simulink model "HCO_two_motor_neurons_mod"  (R2022a)
settings: Solver=VariableStepAuto  StartTime=0.0  StopTime=20  RelTol=1e-3
undefined symbols (not defined in the file or in its folder): bar_amp, buff_amp, dfm, dfm_mod, dgsm_g, dhco, dsm, dsm_mod, dsp, dsp_mod, dsyn, dup, dup_mod, gfm, gfm_mod, ghco, gsm, gsm_mod, gsp, gsp_mod, gsyn, gup, gup_mod, Iapp, Iapp_mod, max_torque, noisePwr, rflx_g, sampleTime, sr_gain, X, Y, Z
libraries: sm_lib x12, simulink x8, nesl_utility x8
settings Model: Creator=chris  LastModifiedBy=chris

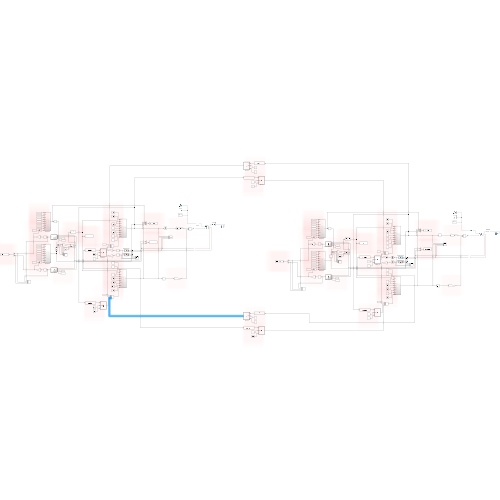
[thumbnail: Simulink's stored preview of the top-level diagram]
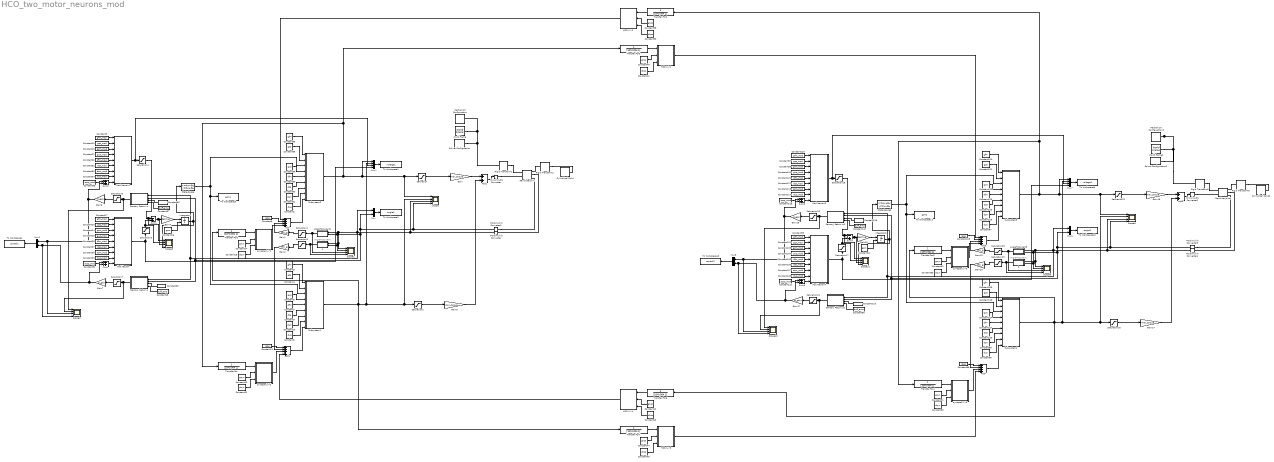
== system HCO_two_motor_neurons_mod ==
  note: AngleToCurrent
  note: AngleToCurrent
  1 : MATLAB Function  TreatAsAtomicUnit=on
  3 : MATLAB Function  TreatAsAtomicUnit=on
  Add{,1,6..7} (4 alike) : Sum  Inputs=++++
  Add2 : Sum
  Add8 : Sum
  AngleToCurrent1 : MATLAB Function  TreatAsAtomicUnit=on
  AngleToCurrent3 : MATLAB Function  TreatAsAtomicUnit=on
  Constant{1..2,87,98} (4 alike) : Constant  Value=dup
  Constant{10,61,88,126} (4 alike) : Constant  Value=dsm
  Constant{21,25,100,104} (4 alike) : Constant  Value=gup_mod
  Constant{22,26,101,105} (4 alike) : Constant  Value=dfm_mod
  Constant{19,23,97,102} (4 alike) : Constant  Value=gsp_mod
  Constant{20,24,99,103} (4 alike) : Constant  Value=gsm_mod
  Constant{27,32,106,112} (4 alike) : Constant  Value=dsp_mod
  Constant{28,33,107,113} (4 alike) : Constant  Value=dsm_mod
  Constant{29,34,108,114} (4 alike) : Constant  Value=dup_mod
  Constant{3,55,109,120} (4 alike) : Constant  Value=gfm
  Constant{8,11,89,128} (4 alike) : Constant  Value=Iapp
  Constant{30,36,110,116} (4 alike) : Constant  Value=bar_amp
  Constant{31,35,111,115} (4 alike) : Constant  Value=Iapp_mod
  Constant{18,37,96,117} (4 alike) : Constant  Value=buff_amp
  Constant{4,56,118,121} (4 alike) : Constant  Value=gsp
  Constant{5,17,95,119} (4 alike) : Constant  Value=gfm_mod
  Constant{12,15,90,93} (4 alike) : Constant  Value=dsyn
  Constant{6,58,122,124} (4 alike) : Constant  Value=gup
  Constant{7,59,123,127} (4 alike) : Constant  Value=dfm
  Constant{9,60,125,129} (4 alike) : Constant  Value=dsp
  Constant{13..14,91..92} (4 alike) : Constant  Value=gsyn
  Constant16 : Constant  Value=gsm
  Constant{38,40,42,44} (4 alike) : Constant  Value=ghco
  Constant{39,41,43,45} (4 alike) : Constant  Value=dhco
  Constant94 : Constant  Value=gsm
  Cylindrical Solid : sm_lib/Body Elements/Cylindrical Solid  GraphicAmbientColor=[0.15 0.15 0.15 1.0]  BasedOnType=Density  CenterOfMass=[0 0 0]  CenterOfMassUnits=m  GraphicDiffuseColor=[0.5 0.5 0.5]  CylinderLength=0.5  CylinderLengthUnits=m  CylinderRadius=0.05  CylinderRadiusUnits=m  Density=1000  DensityUnits=kg/m^3  DoExposeReferenceFrame=on  GraphicEmissiveColor=[0.0 0.0 0.0 1.0]  ExportEntireGeometry=off  SerializedFrames=<Frames/>  MarkerShape=Sphere  MarkerSize=10  GraphicType=FromGeometry  InertiaType=CalculateFromGeometry  Mass=1  MassUnits=kg  MomentsOfInertia=[1 1 1]  MomentsOfInertiaUnits=kg*m^2  GraphicOpacity=1.0  ProductsOfInertia=[0 0 0]  ProductsOfInertiaUnits=kg*m^2  GraphicShininess=75  GraphicSpecularColor=[0.5 0.5 0.5 1.0]  GraphicVisPropType=SimpleVisualProperties
  Cylindrical Solid2 : sm_lib/Body Elements/Cylindrical Solid  GraphicAmbientColor=[0.15 0.15 0.15 1.0]  BasedOnType=Density  CenterOfMass=[0 0 0]  CenterOfMassUnits=m  GraphicDiffuseColor=[0.5 0.5 0.5]  CylinderLength=0.5  CylinderLengthUnits=m  CylinderRadius=0.05  CylinderRadiusUnits=m  Density=1000  DensityUnits=kg/m^3  DoExposeReferenceFrame=on  GraphicEmissiveColor=[0.0 0.0 0.0 1.0]  ExportEntireGeometry=off  SerializedFrames=<Frames/>  MarkerShape=Sphere  MarkerSize=10  GraphicType=FromGeometry  InertiaType=CalculateFromGeometry  Mass=1  MassUnits=kg  MomentsOfInertia=[1 1 1]  MomentsOfInertiaUnits=kg*m^2  GraphicOpacity=1.0  ProductsOfInertia=[0 0 0]  ProductsOfInertiaUnits=kg*m^2  GraphicShininess=75  GraphicSpecularColor=[0.5 0.5 0.5 1.0]  GraphicVisPropType=SimpleVisualProperties
  Gain : Gain  Gain=max_torque
  Gain{1..2,19..20} (4 alike) : Gain  Gain=rflx_g
  Gain14 : Gain  Gain=-max_torque
  Gain15 : Gain  Gain=dgsm_g
  Gain{6..7,16..17} (4 alike) : Gain  Gain=sr_gain
  Gain18 : Gain  Gain=max_torque
  Gain3 : Gain  Gain=-max_torque
  Gain4 : Gain  Gain=dgsm_g
  HCO 1->1 : MATLAB Function  TreatAsAtomicUnit=on
  HCO 1->2 : MATLAB Function  TreatAsAtomicUnit=on
  HCO 1->3 : MATLAB Function  TreatAsAtomicUnit=on
  HCO 1->4 : MATLAB Function  TreatAsAtomicUnit=on
  Integrator : Integrator  InitialConditionSource=external
  Integrator2 : Integrator  InitialConditionSource=external
  Mechanism Configuration : sm_lib/Utilities/Mechanism Configuration  UniformGravity=Constant  GravityVector=[0 0 -9.80665]  GravityUnits=m/s^2  LinearizationDelta=0.001  JointModeTransitionNonlinearIterations=2
  Mechanism Configuration2 : sm_lib/Utilities/Mechanism Configuration  UniformGravity=Constant  GravityVector=[0 0 -9.80665]  GravityUnits=m/s^2  LinearizationDelta=0.001  JointModeTransitionNonlinearIterations=2
  Mod Neuron : Subsystem
  Mod Neuron1 : Subsystem
  Mod Neuron4 : Subsystem
  Mod Neuron5 : Subsystem
  Mux{,2,6,8} (4 alike) : Mux  Inputs=2
  Mux1 : Mux
  Mux7 : Mux
  PS-Simulink Converter{,1,4..5} (4 alike) : nesl_utility/PS-Simulink Converter  PhysicalDomain=network_engine_domain  SubClassName=ps_output  LeftPortType=input  RightPortType=output  PseudoPeriodic=off  Frequencies=[]  VectorFormat=inherit  Unit=inherit  AffineConversion=off
      settings: SourceProductBaseCode=SS,PW,VE
  Revolute Joint : sm_lib/Joints/Revolute Joint  JointMode=Normal  SenseConstraintForce=off  SenseConstraintForceX=off  SenseConstraintForceY=off  SenseConstraintForceZ=off  SenseConstraintTorque=off  SenseConstraintTorqueX=off  SenseConstraintTorqueY=off  SenseConstraintTorqueZ=off  SenseTotalForce=off  SenseTotalForceX=off  SenseTotalForceY=off  SenseTotalForceZ=off  SenseTotalTorque=off  SenseTotalTorqueX=off  SenseTotalTorqueY=off  SenseTotalTorqueZ=off  CompositeWrenchDir=FollowerOnBase  CompositeWrenchFrame=BaseFrame  EquilibriumPosition=0  EquilibriumPositionUnits=deg  SpringStiffness=0.0  SpringStiffnessUnits=N*m/deg  DampingCoefficient=0.01  DampingCoefficientUnits=N*m/(deg/s)  TorqueActuationMode=InputTorque  MotionActuationMode=ComputedMotion  SensePosition=on  SenseVelocity=on  SenseAcceleration=off  SenseTorqueForce=off  SenseLowerLimitTorqueForce=off  SenseUpperLimitTorqueForce=off  LowerLimitSpecify=off  LowerLimitBound=-90  LowerLimitBoundUnits=deg  LowerLimitStiffness=1e4  LowerLimitStiffnessUnits=N*m/deg  LowerLimitDamping=10  LowerLimitDampingUnits=N*m/(deg/s)  LowerLimitTransitionRegionWidth=0.1  LowerLimitTransitionRegionWidthUnits=deg  UpperLimitSpecify=off  UpperLimitBound=90  UpperLimitBoundUnits=deg  UpperLimitStiffness=1e4  UpperLimitStiffnessUnits=N*m/deg  UpperLimitDamping=10  UpperLimitDampingUnits=N*m/(deg/s)  UpperLimitTransitionRegionWidth=0.1  UpperLimitTransitionRegionWidthUnits=deg  PositionTargetSpecify=on  PositionTargetPriority=High  PositionTargetValue=20  PositionTargetValueUnits=deg  VelocityTargetSpecify=off  VelocityTargetPriority=High  VelocityTargetValue=0  VelocityTargetValueUnits=deg/s
  Revolute Joint2 : sm_lib/Joints/Revolute Joint  JointMode=Normal  SenseConstraintForce=off  SenseConstraintForceX=off  SenseConstraintForceY=off  SenseConstraintForceZ=off  SenseConstraintTorque=off  SenseConstraintTorqueX=off  SenseConstraintTorqueY=off  SenseConstraintTorqueZ=off  SenseTotalForce=off  SenseTotalForceX=off  SenseTotalForceY=off  SenseTotalForceZ=off  SenseTotalTorque=off  SenseTotalTorqueX=off  SenseTotalTorqueY=off  SenseTotalTorqueZ=off  CompositeWrenchDir=FollowerOnBase  CompositeWrenchFrame=BaseFrame  EquilibriumPosition=0  EquilibriumPositionUnits=deg  SpringStiffness=0.0  SpringStiffnessUnits=N*m/deg  DampingCoefficient=0.01  DampingCoefficientUnits=N*m/(deg/s)  TorqueActuationMode=InputTorque  MotionActuationMode=ComputedMotion  SensePosition=on  SenseVelocity=on  SenseAcceleration=off  SenseTorqueForce=off  SenseLowerLimitTorqueForce=off  SenseUpperLimitTorqueForce=off  LowerLimitSpecify=off  LowerLimitBound=-90  LowerLimitBoundUnits=deg  LowerLimitStiffness=1e4  LowerLimitStiffnessUnits=N*m/deg  LowerLimitDamping=10  LowerLimitDampingUnits=N*m/(deg/s)  LowerLimitTransitionRegionWidth=0.1  LowerLimitTransitionRegionWidthUnits=deg  UpperLimitSpecify=off  UpperLimitBound=90  UpperLimitBoundUnits=deg  UpperLimitStiffness=1e4  UpperLimitStiffnessUnits=N*m/deg  UpperLimitDamping=10  UpperLimitDampingUnits=N*m/(deg/s)  UpperLimitTransitionRegionWidth=0.1  UpperLimitTransitionRegionWidthUnits=deg  PositionTargetSpecify=on  PositionTargetPriority=High  PositionTargetValue=20  PositionTargetValueUnits=deg  VelocityTargetSpecify=off  VelocityTargetPriority=High  VelocityTargetValue=0  VelocityTargetValueUnits=deg/s
  Rigid Transform1 : sm_lib/Frames and Transforms/Rigid Transform  TranslationMethod=None  TranslationStandardOffset=0.25  TranslationLengthUnit=m  TranslationStandardAxis=+X  TranslationCartesianOffset=[0 0 0]  TranslationROffset=0  TranslationROffsetUnits=m  TranslationZOffset=0  TranslationZOffsetUnits=m  TranslationThetaOffset=0  TranslationThetaOffsetUnits=deg  RotationMethod=RotationSequence  RotationAngleUnits=deg  RotationStandardAxis=+Y  RotationAngle=90  RotationArbitraryAxis=[0 0 1]  FollAlignAxisA=+X  BaseAlignAxisA=+Y  FollAlignAxisB=+Y  BaseAlignAxisB=+Z  RotationSequenceAxes=FollowerAxes  RotationSequence=XYX  RotationSequenceAngles=[0 90 90]  RotationSequenceAnglesUnits=deg  RotationMatrix=[1 0 0; 0 1 0; 0 0 1]
  Rigid Transform2 : sm_lib/Frames and Transforms/Rigid Transform  TranslationMethod=StandardAxis  TranslationStandardOffset=.25  TranslationLengthUnit=m  TranslationStandardAxis=+X  TranslationCartesianOffset=[0 0 0]  TranslationROffset=0  TranslationROffsetUnits=m  TranslationZOffset=0  TranslationZOffsetUnits=m  TranslationThetaOffset=0  TranslationThetaOffsetUnits=deg  RotationMethod=RotationSequence  RotationAngleUnits=deg  RotationStandardAxis=+Z  RotationAngle=90  RotationArbitraryAxis=[0 0 1]  FollAlignAxisA=+X  BaseAlignAxisA=+Y  FollAlignAxisB=+Y  BaseAlignAxisB=+Z  RotationSequenceAxes=FollowerAxes  RotationSequence=XYX  RotationSequenceAngles=[0 90 0]  RotationSequenceAnglesUnits=deg  RotationMatrix=[1 0 0; 0 1 0; 0 0 1]
  Rigid Transform5 : sm_lib/Frames and Transforms/Rigid Transform  TranslationMethod=None  TranslationStandardOffset=0.25  TranslationLengthUnit=m  TranslationStandardAxis=+X  TranslationCartesianOffset=[0 0 0]  TranslationROffset=0  TranslationROffsetUnits=m  TranslationZOffset=0  TranslationZOffsetUnits=m  TranslationThetaOffset=0  TranslationThetaOffsetUnits=deg  RotationMethod=RotationSequence  RotationAngleUnits=deg  RotationStandardAxis=+Y  RotationAngle=90  RotationArbitraryAxis=[0 0 1]  FollAlignAxisA=+X  BaseAlignAxisA=+Y  FollAlignAxisB=+Y  BaseAlignAxisB=+Z  RotationSequenceAxes=FollowerAxes  RotationSequence=XYX  RotationSequenceAngles=[0 90 90]  RotationSequenceAnglesUnits=deg  RotationMatrix=[1 0 0; 0 1 0; 0 0 1]
  Rigid Transform6 : sm_lib/Frames and Transforms/Rigid Transform  TranslationMethod=StandardAxis  TranslationStandardOffset=.25  TranslationLengthUnit=m  TranslationStandardAxis=+X  TranslationCartesianOffset=[0 0 0]  TranslationROffset=0  TranslationROffsetUnits=m  TranslationZOffset=0  TranslationZOffsetUnits=m  TranslationThetaOffset=0  TranslationThetaOffsetUnits=deg  RotationMethod=RotationSequence  RotationAngleUnits=deg  RotationStandardAxis=+Z  RotationAngle=90  RotationArbitraryAxis=[0 0 1]  FollAlignAxisA=+X  BaseAlignAxisA=+Y  FollAlignAxisB=+Y  BaseAlignAxisB=+Z  RotationSequenceAxes=FollowerAxes  RotationSequence=XYX  RotationSequenceAngles=[0 90 0]  RotationSequenceAnglesUnits=deg  RotationMatrix=[1 0 0; 0 1 0; 0 0 1]
  Saturation{,1..7,16..23} (16 alike) : Saturate  UpperLimit=1.0  LowerLimit=0.0
  Scope{,1..3,8..11} (8 alike) : Scope  NumInputPorts=4
  Sensory Return m : MATLAB Function  TreatAsAtomicUnit=on
  Sensory Return m2 : MATLAB Function  TreatAsAtomicUnit=on
  Sensory Return p : MATLAB Function  TreatAsAtomicUnit=on
  Sensory Return p2 : MATLAB Function  TreatAsAtomicUnit=on
  Simulink-PS Converter : nesl_utility/Simulink-PS Converter  PhysicalDomain=network_engine_domain  SubClassName=ps_input  LeftPortType=input  RightPortType=output  PseudoPeriodic=off  Frequencies=[]  NoiseDistribution=none  NoiseParameters=[]  Unit=1  AffineConversion=off  FilteringAndDerivatives=provide  SimscapeFilterOrder=1  InputFilterTimeConstant=0.001  UdotUserProvided=0
      settings: SourceProductBaseCode=SS,PW,VE
  Simulink-PS Converter2 : nesl_utility/Simulink-PS Converter  PhysicalDomain=network_engine_domain  SubClassName=ps_input  LeftPortType=input  RightPortType=output  PseudoPeriodic=off  Frequencies=[]  NoiseDistribution=none  NoiseParameters=[]  Unit=1  AffineConversion=off  FilteringAndDerivatives=provide  SimscapeFilterOrder=1  InputFilterTimeConstant=0.001  UdotUserProvided=0
      settings: SourceProductBaseCode=SS,PW,VE
  Solver Configuration : nesl_utility/Solver Configuration  PhysicalDomain=network_engine_domain  SubClassName=solver  LeftPortType=input  RightPortType=generic  Tones=[]  Harmonics=[]  SimulateNoise=off  Profile=off  UseLocalSampling=off  EnableSwitchedLinearOptims=on  FrequencyDomain=off  UseCCode=off  RelTol=0.001  AbsTol=1e-06  MinStep=1e-09  ToWorkspace=off  RevertToSquareIcSolve=off  NumHomotopyIterations=100  PhasorMode=off  PhasorModeNumHarmonics=1  IndexReductionMethod=DerivativeReplacement  DoDC=off  ResidualTolerance=1e-09  UseLocalSolver=off  LocalSolverChoice=NE_BACKWARD_EULER_ADVANCER  LocalSolverSampleTime=0.001  DoFixedCost=off  MaxNonlinIter=3  MaxModeIter=2  ComputeImpulses=off  ImpulseIterations=2  LinearAlgebra=auto  LinearAlgebraNumThread=0  EquationFormulation=NE_TIME_EF  DelaysMemoryBudget=1024  AutomaticFiltering=on  FilteringTimeConstant=0.001  PartitionStorageMethod=AS_NEEDED  PartitionMemoryBudget=1024  PartitionMethod=ROBUST
      settings: SourceProductBaseCode=SS,PW,VE
  Solver Configuration2 : nesl_utility/Solver Configuration  PhysicalDomain=network_engine_domain  SubClassName=solver  LeftPortType=input  RightPortType=generic  Tones=[]  Harmonics=[]  SimulateNoise=off  Profile=off  UseLocalSampling=off  EnableSwitchedLinearOptims=on  FrequencyDomain=off  UseCCode=off  RelTol=0.001  AbsTol=1e-06  MinStep=1e-09  ToWorkspace=off  RevertToSquareIcSolve=off  NumHomotopyIterations=100  PhasorMode=off  PhasorModeNumHarmonics=1  IndexReductionMethod=DerivativeReplacement  DoDC=off  ResidualTolerance=1e-09  UseLocalSolver=off  LocalSolverChoice=NE_BACKWARD_EULER_ADVANCER  LocalSolverSampleTime=0.001  DoFixedCost=off  MaxNonlinIter=3  MaxModeIter=2  ComputeImpulses=off  ImpulseIterations=2  LinearAlgebra=auto  LinearAlgebraNumThread=0  EquationFormulation=NE_TIME_EF  DelaysMemoryBudget=1024  AutomaticFiltering=on  FilteringTimeConstant=0.001  PartitionStorageMethod=AS_NEEDED  PartitionMemoryBudget=1024  PartitionMethod=ROBUST
      settings: SourceProductBaseCode=SS,PW,VE
  State-Space : StateSpace  A=-10  B=10  D=0  InitialCondition=gsm
  State-Space2 : StateSpace  A=-10  B=10  D=0  InitialCondition=gsm
  Subsystem1 : Subsystem
  Subsystem4 : Subsystem
  Subsystem5 : Subsystem
  Subsystem6 : Subsystem
  Sum{,2,6,8} (4 alike) : Sum
  Sum1 : Sum  Inputs=-+
  Sum7 : Sum  Inputs=-+
  To Workspace1 : ToWorkspace  VariableName=voltage1  SaveFormat=Structure With Time  SampleTime=sampleTime
  To Workspace10 : ToWorkspace  VariableName=angle2  SaveFormat=Structure With Time  SampleTime=sampleTime
  To Workspace11 : ToWorkspace  VariableName=gsm2  SaveFormat=Structure With Time  SampleTime=sampleTime
  To Workspace12 : ToWorkspace  VariableName=control2  SaveFormat=Structure With Time  SampleTime=sampleTime
  To Workspace2 : ToWorkspace  VariableName=angle1  SaveFormat=Structure With Time  SampleTime=sampleTime
  To Workspace3 : ToWorkspace  VariableName=gsm1  SaveFormat=Structure With Time  SampleTime=sampleTime
  To Workspace4 : ToWorkspace  VariableName=control1  SaveFormat=Structure With Time  SampleTime=sampleTime
  To Workspace9 : ToWorkspace  VariableName=voltage2  SaveFormat=Structure With Time  SampleTime=sampleTime
  Transfer Fcn{,1..7} (8 alike) : TransferFcn  Denominator=[10*0.004 1]
  World Frame : sm_lib/Frames and Transforms/World Frame
  World Frame2 : sm_lib/Frames and Transforms/World Frame
  synapse 1->1 : MATLAB Function  TreatAsAtomicUnit=on
  synapse 1->2 : MATLAB Function  TreatAsAtomicUnit=on
  synapse 1->5 : MATLAB Function  TreatAsAtomicUnit=on
  synapse 1->6 : MATLAB Function  TreatAsAtomicUnit=on
  wires:
  Subsystem6/1(V) -> Scope/1, Saturation/1, Mux1/1, Transfer Fcn3/1, Transfer Fcn/1
  Constant60/1 -> Subsystem6/6(dsp)
  Constant1/1 -> Subsystem6/8(dup)
  Constant59/1 -> Subsystem6/5(dfm)
  Constant61/1 -> Subsystem6/7(dsm)
  Constant56/1 -> Subsystem6/2(gsp)
  Constant58/1 -> Subsystem6/4(gup)
  Constant55/1 -> Subsystem6/1(gfm)
  Saturation/1 -> Gain/1
  Add/1 -> Subsystem6/9(Iapp)
  Mux/1 -> To Workspace2/1
  PS-Simulink Converter1/1 -> Scope/4, Mux/2, Scope1/2, 1/2(du), AngleToCurrent1/2(du), Sensory Return m/2(du), Sensory Return p/2(du)
  Constant9/1 -> Subsystem1/6(dsp)
  Constant11/1 -> Add1/1
  Constant10/1 -> Subsystem1/7(dsm)
  Constant3/1 -> Subsystem1/1(gfm)
  Constant4/1 -> Subsystem1/2(gsp)
  Constant7/1 -> Subsystem1/5(dfm)
  Add1/1 -> Subsystem1/9(Iapp)
  Constant6/1 -> Subsystem1/4(gup)
  Constant2/1 -> Subsystem1/8(dup)
  Gain2/1 -> Add1/2
  Subsystem1/1(V) -> Transfer Fcn1/1, Transfer Fcn7/1, Saturation2/1, Scope/2, Mux1/2
  Saturation2/1 -> Gain3/1
  Add2/1 -> Simulink-PS Converter/1
  Gain/1 -> Add2/1
  Gain3/1 -> Add2/2
  synapse 1->2/1(I) -> Add1/3
  Transfer Fcn/1 -> synapse 1->2/1(V)
  Transfer Fcn1/1 -> synapse 1->1/1(V)
  Constant13/1 -> synapse 1->2/2(gsyn)
  Constant12/1 -> synapse 1->2/3(d)
  Constant15/1 -> synapse 1->1/3(d)
  Constant14/1 -> synapse 1->1/2(gsyn)
  Mux1/1 -> To Workspace1/1
  Sum/1 -> Mod Neuron/9(Iapp)
  Constant30/1 -> Sensory Return p/3(bar_amp)
  Constant17/1 -> Mod Neuron/1(gfm)
  Constant23/1 -> Mod Neuron/2(gsp)
  Constant31/1 -> Sum/1
  Constant28/1 -> Mod Neuron/7(dsm)
  Constant26/1 -> Mod Neuron/5(dfm)
  Constant27/1 -> Mod Neuron/6(dsp)
  Constant24/1 -> Mod Neuron/3(gsm)
  Constant25/1 -> Mod Neuron/4(gup)
  Constant29/1 -> Mod Neuron/8(dup)
  PS-Simulink Converter/1 -> Scope/3, Scope1/1, 1/1(u), AngleToCurrent1/1(u), Sensory Return m/1(u), Sensory Return p/1(u), Mux/1
  Constant16/1 -> Integrator/2
  Mod Neuron/1(V) -> Saturation3/1, Mux1/4
  Saturation4/1 -> Scope3/1, Sum1/1
  Saturation3/1 -> Scope3/2, Sum1/2
  Integrator/1 -> State-Space/1, Scope3/4
  State-Space/1 -> Subsystem6/3(gsm), Subsystem1/3(gsm), To Workspace3/1
  Gain4/1 -> Integrator/1
  Sum1/1 -> Scope3/3, Gain4/1
  Sum2/1 -> Mod Neuron1/9(Iapp)
  Constant22/1 -> Mod Neuron1/5(dfm)
  Constant35/1 -> Sum2/1
  Constant21/1 -> Mod Neuron1/4(gup)
  Constant32/1 -> Mod Neuron1/6(dsp)
  Constant20/1 -> Mod Neuron1/3(gsm)
  Constant33/1 -> Mod Neuron1/7(dsm)
  Constant5/1 -> Mod Neuron1/1(gfm)
  Constant19/1 -> Mod Neuron1/2(gsp)
  Constant34/1 -> Mod Neuron1/8(dup)
  Constant36/1 -> Sensory Return m/3(bar_amp)
  Sensory Return m/1(y) -> Scope2/1, Saturation6/1
  Mod Neuron1/1(V) -> Mux1/3, Saturation4/1
  Mux2/1 -> To Workspace4/1
  Saturation1/1 -> Gain1/1
  Saturation5/1 -> Gain2/1
  Gain6/1 -> Scope2/3, Mux2/1, Sum2/2
  Sensory Return p/1(y) -> Scope2/2, Saturation7/1
  Gain7/1 -> Mux2/2, Scope2/4, Sum/2
  AngleToCurrent1/1(y) -> Saturation1/1, Scope1/3
  1/1(y) -> Scope1/4, Saturation5/1
  Saturation6/1 -> Gain6/1
  Saturation7/1 -> Gain7/1
  Constant18/1 -> Sensory Return p/4(buff_amp)
  Constant37/1 -> Sensory Return m/4(buff_amp)
  Constant120/1 -> Subsystem5/1(gfm)
  Constant105/1 -> Mod Neuron4/5(dfm)
  Constant121/1 -> Subsystem5/2(gsp)
  Saturation22/1 -> Gain18/1
  Constant122/1 -> Subsystem5/4(gup)
  Mux6/1 -> To Workspace10/1
  Constant126/1 -> Subsystem5/7(dsm)
  Add6/1 -> Subsystem5/9(Iapp)
  Constant118/1 -> Subsystem4/2(gsp)
  State-Space2/1 -> To Workspace11/1, Subsystem4/3(gsm), Subsystem5/3(gsm)
  Gain20/1 -> Add7/2
  Constant89/1 -> Add7/1
  Transfer Fcn4/1 -> synapse 1->6/1(V)
  Constant90/1 -> synapse 1->6/3(d)
  Constant92/1 -> synapse 1->5/2(gsyn)
  Constant91/1 -> synapse 1->6/2(gsyn)
  PS-Simulink Converter5/1 -> Sensory Return p2/2(du), Sensory Return m2/2(du), AngleToCurrent3/2(du), 3/2(du), Scope9/2, Mux6/2, Scope8/4
  Sum6/1 -> Mod Neuron4/9(Iapp)
  Constant93/1 -> synapse 1->5/3(d)
  Saturation16/1 -> Gain14/1
  Saturation17/1 -> Sum7/2, Scope11/2
  Constant123/1 -> Subsystem5/5(dfm)
  Gain14/1 -> Add8/2
  Constant124/1 -> Subsystem4/4(gup)
  Constant102/1 -> Mod Neuron4/2(gsp)
  Constant104/1 -> Mod Neuron4/4(gup)
  Constant111/1 -> Sum6/1
  Constant103/1 -> Mod Neuron4/3(gsm)
  Mux7/1 -> To Workspace9/1
  Constant110/1 -> Sensory Return p2/3(bar_amp)
  Constant127/1 -> Subsystem4/5(dfm)
  Integrator2/1 -> Scope11/4, State-Space2/1
  Constant94/1 -> Integrator2/2
  Constant108/1 -> Mod Neuron4/8(dup)
  PS-Simulink Converter4/1 -> Mux6/1, Sensory Return p2/1(u), Sensory Return m2/1(u), AngleToCurrent3/1(u), 3/1(u), Scope9/1, Scope8/3
  Subsystem4/1(V) -> Transfer Fcn6/1, Mux7/2, Scope8/2, Saturation16/1, Transfer Fcn5/1
  Sensory Return m2/1(y) -> Saturation20/1, Scope10/1
  Constant97/1 -> Mod Neuron5/2(gsp)
  Constant116/1 -> Sensory Return m2/3(bar_amp)
  Gain15/1 -> Integrator2/1
  Sum7/1 -> Gain15/1, Scope11/3
  Subsystem5/1(V) -> Transfer Fcn2/1, Transfer Fcn4/1, Mux7/1, Saturation22/1, Scope8/1
  Add8/1 -> Simulink-PS Converter2/1
  Constant109/1 -> Subsystem4/1(gfm)
  Constant98/1 -> Subsystem4/8(dup)
  Constant101/1 -> Mod Neuron5/5(dfm)
  Add7/1 -> Subsystem4/9(Iapp)
  Sensory Return p2/1(y) -> Saturation21/1, Scope10/2
  Gain16/1 -> Sum8/2, Mux8/1, Scope10/3
  Constant115/1 -> Sum8/1
  Saturation23/1 -> Gain19/1
  Constant99/1 -> Mod Neuron5/3(gsm)
  Constant106/1 -> Mod Neuron4/6(dsp)
  Saturation19/1 -> Gain20/1
  Mod Neuron5/1(V) -> Saturation18/1, Mux7/3
  Constant113/1 -> Mod Neuron5/7(dsm)
  Constant114/1 -> Mod Neuron5/8(dup)
  Constant119/1 -> Mod Neuron5/1(gfm)
  Mux8/1 -> To Workspace12/1
  AngleToCurrent3/1(y) -> Scope9/3, Saturation23/1
  Saturation20/1 -> Gain16/1
  Gain17/1 -> Sum6/2, Scope10/4, Mux8/2
  Constant129/1 -> Subsystem4/6(dsp)
  Saturation18/1 -> Sum7/1, Scope11/1
  synapse 1->6/1(I) -> Add7/3
  Constant96/1 -> Sensory Return p2/4(buff_amp)
  Transfer Fcn5/1 -> synapse 1->5/1(V)
  Constant100/1 -> Mod Neuron5/4(gup)
  Constant107/1 -> Mod Neuron4/7(dsm)
  Saturation21/1 -> Gain17/1
  Constant112/1 -> Mod Neuron5/6(dsp)
  Gain18/1 -> Add8/1
  Mod Neuron4/1(V) -> Mux7/4, Saturation17/1
  Sum8/1 -> Mod Neuron5/9(Iapp)
  Constant88/1 -> Subsystem4/7(dsm)
  Constant95/1 -> Mod Neuron4/1(gfm)
  3/1(y) -> Saturation19/1, Scope9/4
  Constant117/1 -> Sensory Return m2/4(buff_amp)
  Constant87/1 -> Subsystem5/8(dup)
  Constant125/1 -> Subsystem5/6(dsp)
  Transfer Fcn7/1 -> HCO 1->3/1(V)
  Constant44/1 -> HCO 1->3/2(gsyn)
  Constant45/1 -> HCO 1->3/3(d)
  Transfer Fcn6/1 -> HCO 1->4/1(V)
  Constant43/1 -> HCO 1->4/3(d)
  Constant42/1 -> HCO 1->4/2(gsyn)
  Transfer Fcn3/1 -> HCO 1->1/1(V)
  Constant40/1 -> HCO 1->1/2(gsyn)
  Constant41/1 -> HCO 1->1/3(d)
  Transfer Fcn2/1 -> HCO 1->2/1(V)
  Constant39/1 -> HCO 1->2/3(d)
  Constant38/1 -> HCO 1->2/2(gsyn)
  synapse 1->1/1(I) -> Add/4
  Gain1/1 -> Add/3
  Constant8/1 -> Add/2
  HCO 1->2/1(I) -> Add/1
  Gain19/1 -> Add6/3
  synapse 1->5/1(I) -> Add6/4
  Constant128/1 -> Add6/2
  HCO 1->1/1(I) -> Add6/1
  HCO 1->3/1(I) -> Add7/4
  HCO 1->4/1(I) -> Add1/4
  connections:
  Solver Configuration/RConn1 -- Mechanism Configuration/RConn1 -- World Frame/RConn1 -- Rigid Transform1/LConn1
  Rigid Transform1/RConn1 -- Revolute Joint/LConn1
  Simulink-PS Converter/RConn1 -- Revolute Joint/LConn2
  Rigid Transform2/RConn1 -- Cylindrical Solid/RConn1
  Rigid Transform2/LConn1 -- Revolute Joint/RConn1
  Revolute Joint/RConn2 -- PS-Simulink Converter/LConn1
  PS-Simulink Converter1/LConn1 -- Revolute Joint/RConn3
  Mechanism Configuration2/RConn1 -- Rigid Transform5/LConn1 -- Solver Configuration2/RConn1 -- World Frame2/RConn1
  Simulink-PS Converter2/RConn1 -- Revolute Joint2/LConn2
  PS-Simulink Converter5/LConn1 -- Revolute Joint2/RConn3
  Rigid Transform5/RConn1 -- Revolute Joint2/LConn1
  Revolute Joint2/RConn2 -- PS-Simulink Converter4/LConn1
  Rigid Transform6/LConn1 -- Revolute Joint2/RConn1
  Rigid Transform6/RConn1 -- Cylindrical Solid2/RConn1

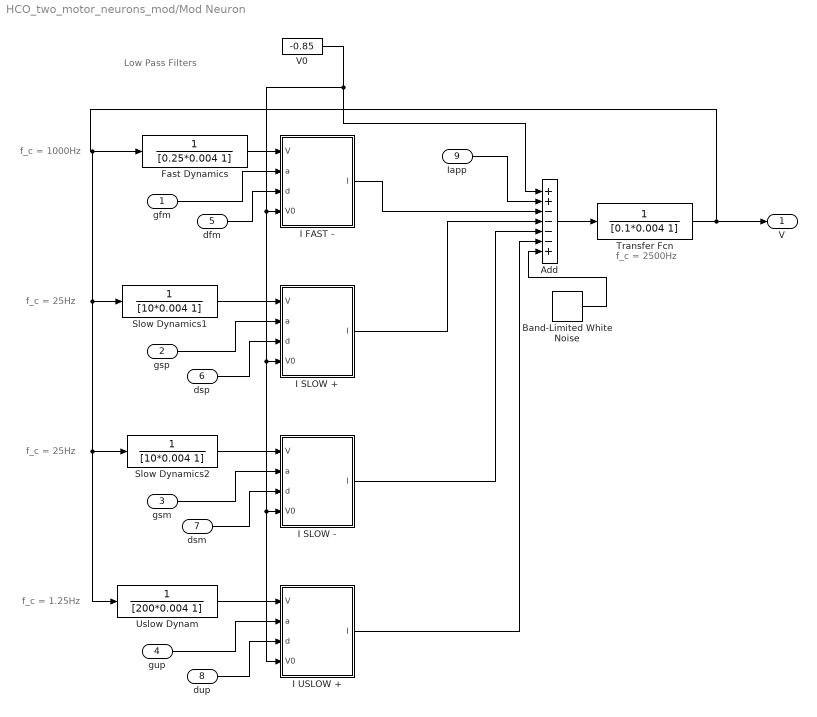
== system HCO_two_motor_neurons_mod/Mod Neuron ==
  note: f_c = 2500Hz
  note: f_c = 1.25Hz
  note: f_c = 25Hz
  note: f_c = 1000Hz
  note: Low Pass Filters
  note: f_c = 25Hz
  gfm : Inport
  gsp : Inport  Port=2
  gsm : Inport  Port=3
  gup : Inport  Port=4
  dfm : Inport  Port=5
  dsp : Inport  Port=6
  dsm : Inport  Port=7
  dup : Inport  Port=8
  Iapp : Inport  Port=9
  Add : Sum  Inputs=++----+
  Band-Limited White Noise : simulink/Sources/Band-Limited White Noise  Cov=[0.0]  Ts=0.1  seed=[23341]
  Fast Dynamics : TransferFcn  Denominator=[0.25*0.004 1]
  I FAST - : MATLAB Function  TreatAsAtomicUnit=on
  I SLOW + : MATLAB Function  TreatAsAtomicUnit=on
  I SLOW - : MATLAB Function  TreatAsAtomicUnit=on
  I USLOW + : MATLAB Function  TreatAsAtomicUnit=on
  Slow Dynamics1 : TransferFcn  Denominator=[10*0.004 1]
  Slow Dynamics2 : TransferFcn  Denominator=[10*0.004 1]
  Transfer Fcn : TransferFcn  Denominator=[0.1*0.004 1]
  Uslow Dynam : TransferFcn  Denominator=[200*0.004 1]
  V0 : Constant  Value=-0.85
  V : Outport
  wires:
  dup/1 -> I USLOW +/3(d)
  gsm/1 -> I SLOW -/2(a)
  dsm/1 -> I SLOW -/3(d)
  gup/1 -> I USLOW +/2(a)
  Iapp/1 -> Add/2
  Uslow Dynam/1 -> I USLOW +/1(V)
  Add/1 -> Transfer Fcn/1
  Slow Dynamics1/1 -> I SLOW +/1(V)
  Slow Dynamics2/1 -> I SLOW -/1(V)
  I FAST -/1(I) -> Add/3
  I USLOW +/1(I) -> Add/6
  V0/1 -> I USLOW +/4(V0), I SLOW -/4(V0), I SLOW +/4(V0), I FAST -/4(V0), Add/1
  dsp/1 -> I SLOW +/3(d)
  gsp/1 -> I SLOW +/2(a)
  dfm/1 -> I FAST -/3(d)
  gfm/1 -> I FAST -/2(a)
  Fast Dynamics/1 -> I FAST -/1(V)
  I SLOW -/1(I) -> Add/5
  Transfer Fcn/1 -> V/1, Uslow Dynam/1, Slow Dynamics2/1, Slow Dynamics1/1, Fast Dynamics/1
  I SLOW +/1(I) -> Add/4
  Band-Limited White Noise/1 -> Add/7

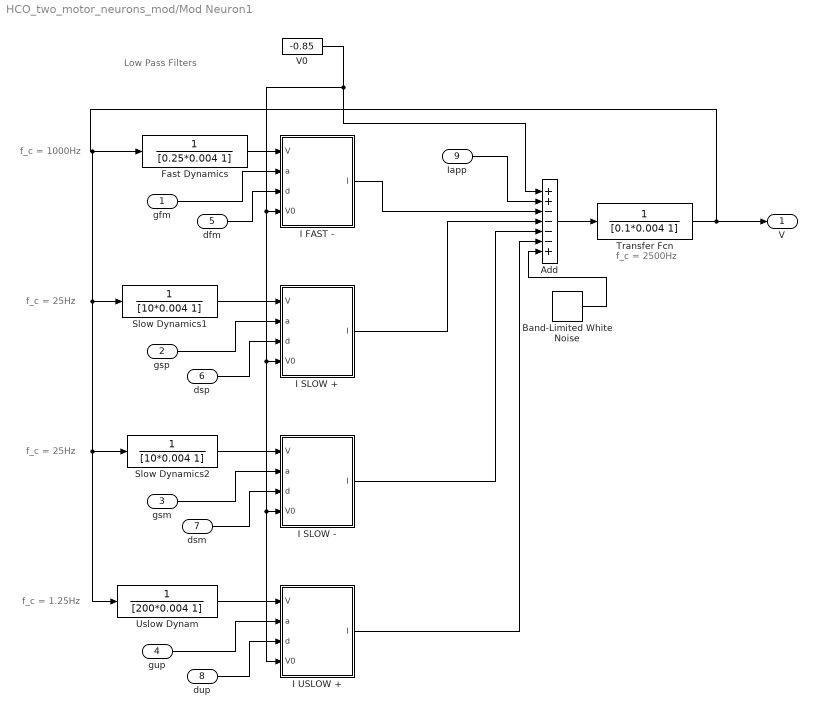
== system HCO_two_motor_neurons_mod/Mod Neuron1 ==
  note: f_c = 2500Hz
  note: f_c = 1.25Hz
  note: f_c = 25Hz
  note: f_c = 1000Hz
  note: Low Pass Filters
  note: f_c = 25Hz
  gfm : Inport
  gsp : Inport  Port=2
  gsm : Inport  Port=3
  gup : Inport  Port=4
  dfm : Inport  Port=5
  dsp : Inport  Port=6
  dsm : Inport  Port=7
  dup : Inport  Port=8
  Iapp : Inport  Port=9
  Add : Sum  Inputs=++----+
  Band-Limited White Noise : simulink/Sources/Band-Limited White Noise  Cov=[0.0]  Ts=0.1  seed=[23341]
  Fast Dynamics : TransferFcn  Denominator=[0.25*0.004 1]
  I FAST - : MATLAB Function  TreatAsAtomicUnit=on
  I SLOW + : MATLAB Function  TreatAsAtomicUnit=on
  I SLOW - : MATLAB Function  TreatAsAtomicUnit=on
  I USLOW + : MATLAB Function  TreatAsAtomicUnit=on
  Slow Dynamics1 : TransferFcn  Denominator=[10*0.004 1]
  Slow Dynamics2 : TransferFcn  Denominator=[10*0.004 1]
  Transfer Fcn : TransferFcn  Denominator=[0.1*0.004 1]
  Uslow Dynam : TransferFcn  Denominator=[200*0.004 1]
  V0 : Constant  Value=-0.85
  V : Outport
  wires:
  dup/1 -> I USLOW +/3(d)
  gsm/1 -> I SLOW -/2(a)
  dsm/1 -> I SLOW -/3(d)
  gup/1 -> I USLOW +/2(a)
  Iapp/1 -> Add/2
  Uslow Dynam/1 -> I USLOW +/1(V)
  Add/1 -> Transfer Fcn/1
  Slow Dynamics1/1 -> I SLOW +/1(V)
  Slow Dynamics2/1 -> I SLOW -/1(V)
  I FAST -/1(I) -> Add/3
  I USLOW +/1(I) -> Add/6
  V0/1 -> I USLOW +/4(V0), I SLOW -/4(V0), I SLOW +/4(V0), I FAST -/4(V0), Add/1
  dsp/1 -> I SLOW +/3(d)
  gsp/1 -> I SLOW +/2(a)
  dfm/1 -> I FAST -/3(d)
  gfm/1 -> I FAST -/2(a)
  Fast Dynamics/1 -> I FAST -/1(V)
  I SLOW -/1(I) -> Add/5
  Transfer Fcn/1 -> V/1, Uslow Dynam/1, Slow Dynamics2/1, Slow Dynamics1/1, Fast Dynamics/1
  I SLOW +/1(I) -> Add/4
  Band-Limited White Noise/1 -> Add/7

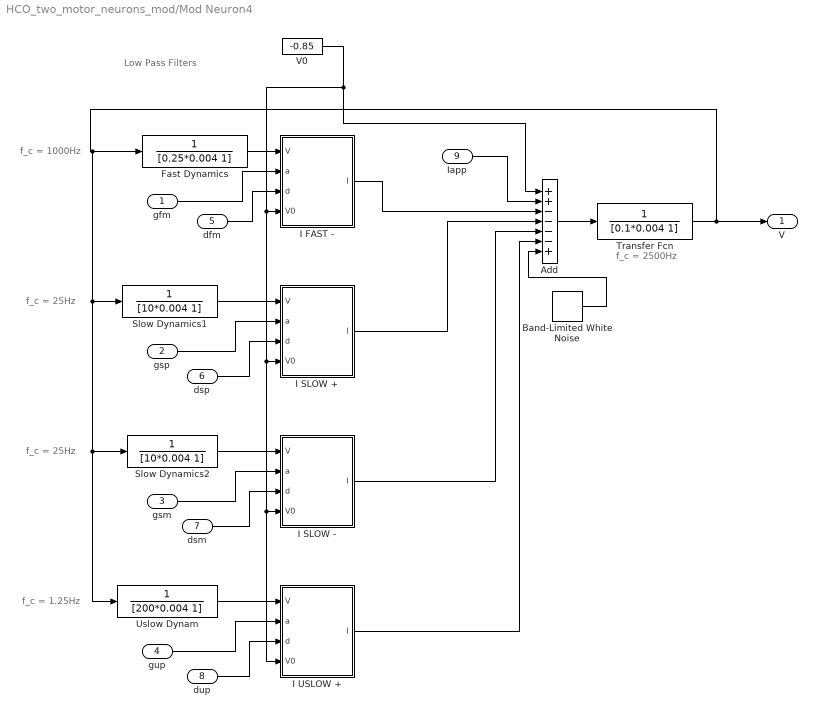
== system HCO_two_motor_neurons_mod/Mod Neuron4 ==
  note: f_c = 25Hz
  note: Low Pass Filters
  note: f_c = 1000Hz
  note: f_c = 25Hz
  note: f_c = 1.25Hz
  note: f_c = 2500Hz
  gfm : Inport
  gsp : Inport  Port=2
  gsm : Inport  Port=3
  gup : Inport  Port=4
  dfm : Inport  Port=5
  dsp : Inport  Port=6
  dsm : Inport  Port=7
  dup : Inport  Port=8
  Iapp : Inport  Port=9
  Add : Sum  Inputs=++----+
  Band-Limited White Noise : simulink/Sources/Band-Limited White Noise  Cov=[0.0]  Ts=0.1  seed=[23341]
  Fast Dynamics : TransferFcn  Denominator=[0.25*0.004 1]
  I FAST - : MATLAB Function  TreatAsAtomicUnit=on
  I SLOW + : MATLAB Function  TreatAsAtomicUnit=on
  I SLOW - : MATLAB Function  TreatAsAtomicUnit=on
  I USLOW + : MATLAB Function  TreatAsAtomicUnit=on
  Slow Dynamics1 : TransferFcn  Denominator=[10*0.004 1]
  Slow Dynamics2 : TransferFcn  Denominator=[10*0.004 1]
  Transfer Fcn : TransferFcn  Denominator=[0.1*0.004 1]
  Uslow Dynam : TransferFcn  Denominator=[200*0.004 1]
  V0 : Constant  Value=-0.85
  V : Outport
  wires:
  Band-Limited White Noise/1 -> Add/7
  I SLOW +/1(I) -> Add/4
  Transfer Fcn/1 -> Fast Dynamics/1, Slow Dynamics1/1, Slow Dynamics2/1, Uslow Dynam/1, V/1
  I SLOW -/1(I) -> Add/5
  Fast Dynamics/1 -> I FAST -/1(V)
  gfm/1 -> I FAST -/2(a)
  dfm/1 -> I FAST -/3(d)
  gsp/1 -> I SLOW +/2(a)
  dsp/1 -> I SLOW +/3(d)
  V0/1 -> Add/1, I FAST -/4(V0), I SLOW +/4(V0), I SLOW -/4(V0), I USLOW +/4(V0)
  I USLOW +/1(I) -> Add/6
  I FAST -/1(I) -> Add/3
  Slow Dynamics2/1 -> I SLOW -/1(V)
  Slow Dynamics1/1 -> I SLOW +/1(V)
  Add/1 -> Transfer Fcn/1
  Uslow Dynam/1 -> I USLOW +/1(V)
  Iapp/1 -> Add/2
  gup/1 -> I USLOW +/2(a)
  dsm/1 -> I SLOW -/3(d)
  gsm/1 -> I SLOW -/2(a)
  dup/1 -> I USLOW +/3(d)

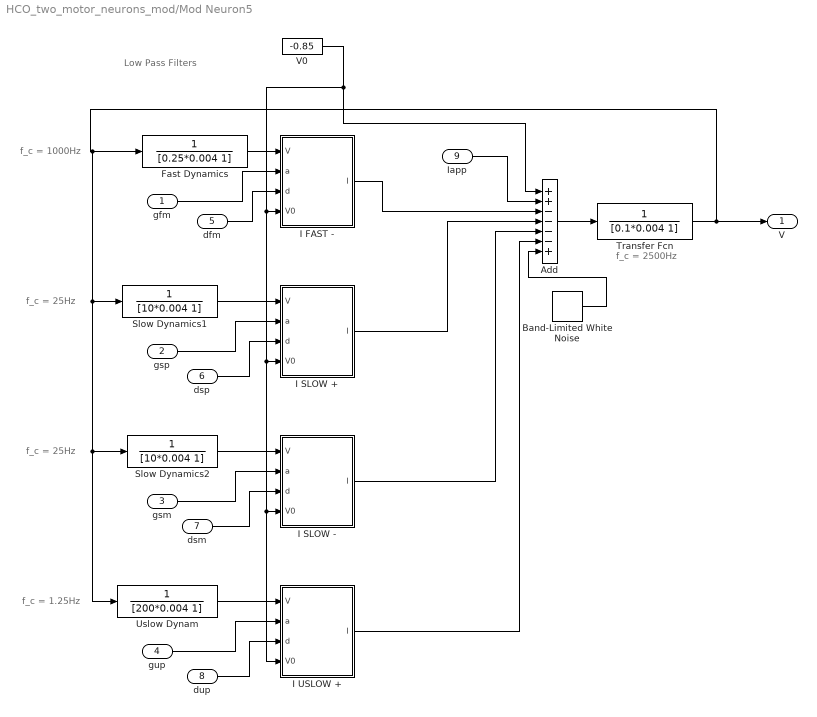
== system HCO_two_motor_neurons_mod/Mod Neuron5 ==
  note: f_c = 25Hz
  note: Low Pass Filters
  note: f_c = 1000Hz
  note: f_c = 25Hz
  note: f_c = 1.25Hz
  note: f_c = 2500Hz
  gfm : Inport
  gsp : Inport  Port=2
  gsm : Inport  Port=3
  gup : Inport  Port=4
  dfm : Inport  Port=5
  dsp : Inport  Port=6
  dsm : Inport  Port=7
  dup : Inport  Port=8
  Iapp : Inport  Port=9
  Add : Sum  Inputs=++----+
  Band-Limited White Noise : simulink/Sources/Band-Limited White Noise  Cov=[0.0]  Ts=0.1  seed=[23341]
  Fast Dynamics : TransferFcn  Denominator=[0.25*0.004 1]
  I FAST - : MATLAB Function  TreatAsAtomicUnit=on
  I SLOW + : MATLAB Function  TreatAsAtomicUnit=on
  I SLOW - : MATLAB Function  TreatAsAtomicUnit=on
  I USLOW + : MATLAB Function  TreatAsAtomicUnit=on
  Slow Dynamics1 : TransferFcn  Denominator=[10*0.004 1]
  Slow Dynamics2 : TransferFcn  Denominator=[10*0.004 1]
  Transfer Fcn : TransferFcn  Denominator=[0.1*0.004 1]
  Uslow Dynam : TransferFcn  Denominator=[200*0.004 1]
  V0 : Constant  Value=-0.85
  V : Outport
  wires:
  Band-Limited White Noise/1 -> Add/7
  I SLOW +/1(I) -> Add/4
  Transfer Fcn/1 -> Fast Dynamics/1, Slow Dynamics1/1, Slow Dynamics2/1, Uslow Dynam/1, V/1
  I SLOW -/1(I) -> Add/5
  Fast Dynamics/1 -> I FAST -/1(V)
  gfm/1 -> I FAST -/2(a)
  dfm/1 -> I FAST -/3(d)
  gsp/1 -> I SLOW +/2(a)
  dsp/1 -> I SLOW +/3(d)
  V0/1 -> Add/1, I FAST -/4(V0), I SLOW +/4(V0), I SLOW -/4(V0), I USLOW +/4(V0)
  I USLOW +/1(I) -> Add/6
  I FAST -/1(I) -> Add/3
  Slow Dynamics2/1 -> I SLOW -/1(V)
  Slow Dynamics1/1 -> I SLOW +/1(V)
  Add/1 -> Transfer Fcn/1
  Uslow Dynam/1 -> I USLOW +/1(V)
  Iapp/1 -> Add/2
  gup/1 -> I USLOW +/2(a)
  dsm/1 -> I SLOW -/3(d)
  gsm/1 -> I SLOW -/2(a)
  dup/1 -> I USLOW +/3(d)

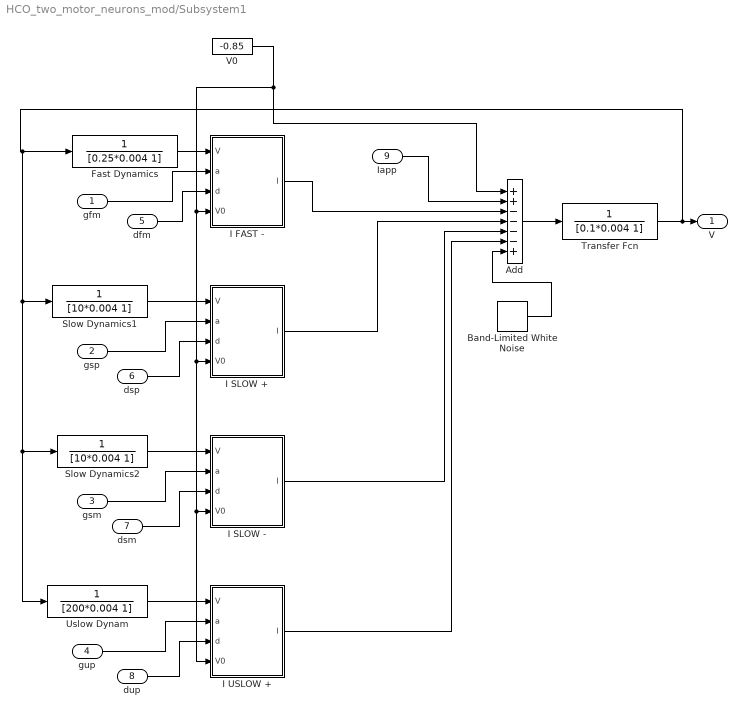
== system HCO_two_motor_neurons_mod/Subsystem1 ==
  gfm : Inport
  gsp : Inport  Port=2
  gsm : Inport  Port=3
  gup : Inport  Port=4
  dfm : Inport  Port=5
  dsp : Inport  Port=6
  dsm : Inport  Port=7
  dup : Inport  Port=8
  Iapp : Inport  Port=9
  Add : Sum  Inputs=++----+
  Band-Limited White Noise : simulink/Sources/Band-Limited White Noise  Cov=[noisePwr]  Ts=0.001  seed=floor(rand(1)*250000)
  Fast Dynamics : TransferFcn  Denominator=[0.25*0.004 1]
  I FAST - : MATLAB Function  TreatAsAtomicUnit=on
  I SLOW + : MATLAB Function  TreatAsAtomicUnit=on
  I SLOW - : MATLAB Function  TreatAsAtomicUnit=on
  I USLOW + : MATLAB Function  TreatAsAtomicUnit=on
  Slow Dynamics1 : TransferFcn  Denominator=[10*0.004 1]
  Slow Dynamics2 : TransferFcn  Denominator=[10*0.004 1]
  Transfer Fcn : TransferFcn  Denominator=[0.1*0.004 1]
  Uslow Dynam : TransferFcn  Denominator=[200*0.004 1]
  V0 : Constant  Value=-0.85
  V : Outport
  wires:
  dup/1 -> I USLOW +/3(d)
  gsm/1 -> I SLOW -/2(a)
  dsm/1 -> I SLOW -/3(d)
  gup/1 -> I USLOW +/2(a)
  Iapp/1 -> Add/2
  Uslow Dynam/1 -> I USLOW +/1(V)
  Add/1 -> Transfer Fcn/1
  Slow Dynamics1/1 -> I SLOW +/1(V)
  Slow Dynamics2/1 -> I SLOW -/1(V)
  I FAST -/1(I) -> Add/3
  I USLOW +/1(I) -> Add/6
  V0/1 -> I USLOW +/4(V0), I SLOW -/4(V0), I SLOW +/4(V0), I FAST -/4(V0), Add/1
  dsp/1 -> I SLOW +/3(d)
  gsp/1 -> I SLOW +/2(a)
  dfm/1 -> I FAST -/3(d)
  gfm/1 -> I FAST -/2(a)
  Fast Dynamics/1 -> I FAST -/1(V)
  I SLOW -/1(I) -> Add/5
  Transfer Fcn/1 -> Uslow Dynam/1, Slow Dynamics2/1, Slow Dynamics1/1, Fast Dynamics/1, V/1
  I SLOW +/1(I) -> Add/4
  Band-Limited White Noise/1 -> Add/7

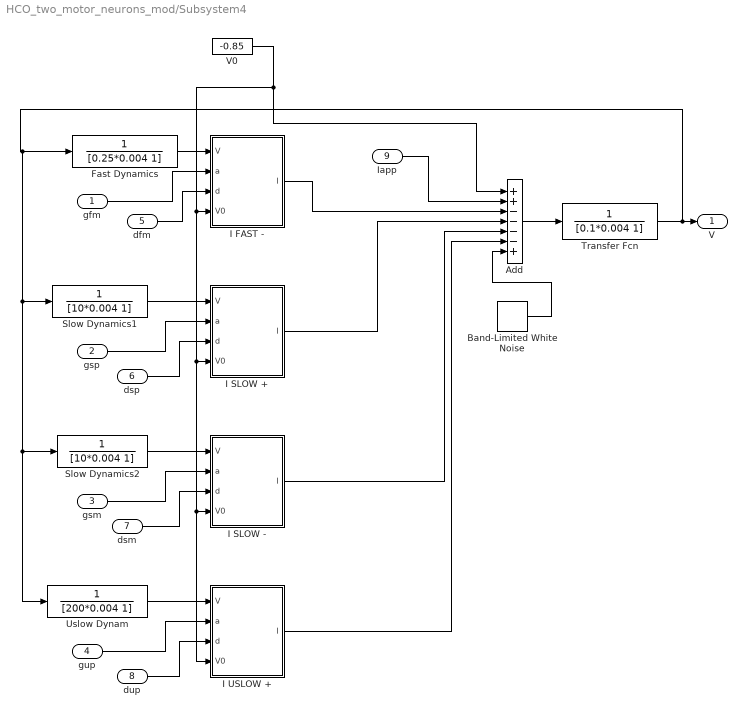
== system HCO_two_motor_neurons_mod/Subsystem4 ==
  gfm : Inport
  gsp : Inport  Port=2
  gsm : Inport  Port=3
  gup : Inport  Port=4
  dfm : Inport  Port=5
  dsp : Inport  Port=6
  dsm : Inport  Port=7
  dup : Inport  Port=8
  Iapp : Inport  Port=9
  Add : Sum  Inputs=++----+
  Band-Limited White Noise : simulink/Sources/Band-Limited White Noise  Cov=[noisePwr]  Ts=0.001  seed=floor(rand(1)*250000)
  Fast Dynamics : TransferFcn  Denominator=[0.25*0.004 1]
  I FAST - : MATLAB Function  TreatAsAtomicUnit=on
  I SLOW + : MATLAB Function  TreatAsAtomicUnit=on
  I SLOW - : MATLAB Function  TreatAsAtomicUnit=on
  I USLOW + : MATLAB Function  TreatAsAtomicUnit=on
  Slow Dynamics1 : TransferFcn  Denominator=[10*0.004 1]
  Slow Dynamics2 : TransferFcn  Denominator=[10*0.004 1]
  Transfer Fcn : TransferFcn  Denominator=[0.1*0.004 1]
  Uslow Dynam : TransferFcn  Denominator=[200*0.004 1]
  V0 : Constant  Value=-0.85
  V : Outport
  wires:
  Band-Limited White Noise/1 -> Add/7
  I SLOW +/1(I) -> Add/4
  Transfer Fcn/1 -> V/1, Fast Dynamics/1, Slow Dynamics1/1, Slow Dynamics2/1, Uslow Dynam/1
  I SLOW -/1(I) -> Add/5
  Fast Dynamics/1 -> I FAST -/1(V)
  gfm/1 -> I FAST -/2(a)
  dfm/1 -> I FAST -/3(d)
  gsp/1 -> I SLOW +/2(a)
  dsp/1 -> I SLOW +/3(d)
  V0/1 -> Add/1, I FAST -/4(V0), I SLOW +/4(V0), I SLOW -/4(V0), I USLOW +/4(V0)
  I USLOW +/1(I) -> Add/6
  I FAST -/1(I) -> Add/3
  Slow Dynamics2/1 -> I SLOW -/1(V)
  Slow Dynamics1/1 -> I SLOW +/1(V)
  Add/1 -> Transfer Fcn/1
  Uslow Dynam/1 -> I USLOW +/1(V)
  Iapp/1 -> Add/2
  gup/1 -> I USLOW +/2(a)
  dsm/1 -> I SLOW -/3(d)
  gsm/1 -> I SLOW -/2(a)
  dup/1 -> I USLOW +/3(d)

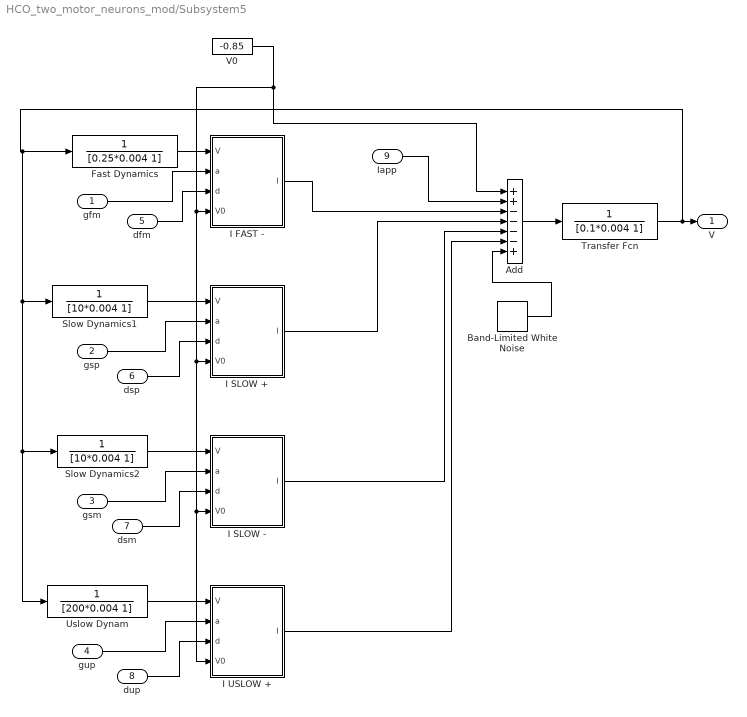
== system HCO_two_motor_neurons_mod/Subsystem5 ==
  gfm : Inport
  gsp : Inport  Port=2
  gsm : Inport  Port=3
  gup : Inport  Port=4
  dfm : Inport  Port=5
  dsp : Inport  Port=6
  dsm : Inport  Port=7
  dup : Inport  Port=8
  Iapp : Inport  Port=9
  Add : Sum  Inputs=++----+
  Band-Limited White Noise : simulink/Sources/Band-Limited White Noise  Cov=[noisePwr]  Ts=0.001  seed=floor(rand(1)*250000)
  Fast Dynamics : TransferFcn  Denominator=[0.25*0.004 1]
  I FAST - : MATLAB Function  TreatAsAtomicUnit=on
  I SLOW + : MATLAB Function  TreatAsAtomicUnit=on
  I SLOW - : MATLAB Function  TreatAsAtomicUnit=on
  I USLOW + : MATLAB Function  TreatAsAtomicUnit=on
  Slow Dynamics1 : TransferFcn  Denominator=[10*0.004 1]
  Slow Dynamics2 : TransferFcn  Denominator=[10*0.004 1]
  Transfer Fcn : TransferFcn  Denominator=[0.1*0.004 1]
  Uslow Dynam : TransferFcn  Denominator=[200*0.004 1]
  V0 : Constant  Value=-0.85
  V : Outport
  wires:
  Band-Limited White Noise/1 -> Add/7
  I SLOW +/1(I) -> Add/4
  Transfer Fcn/1 -> V/1, Fast Dynamics/1, Slow Dynamics1/1, Slow Dynamics2/1, Uslow Dynam/1
  I SLOW -/1(I) -> Add/5
  Fast Dynamics/1 -> I FAST -/1(V)
  gfm/1 -> I FAST -/2(a)
  dfm/1 -> I FAST -/3(d)
  gsp/1 -> I SLOW +/2(a)
  dsp/1 -> I SLOW +/3(d)
  V0/1 -> Add/1, I FAST -/4(V0), I SLOW +/4(V0), I SLOW -/4(V0), I USLOW +/4(V0)
  I USLOW +/1(I) -> Add/6
  I FAST -/1(I) -> Add/3
  Slow Dynamics2/1 -> I SLOW -/1(V)
  Slow Dynamics1/1 -> I SLOW +/1(V)
  Add/1 -> Transfer Fcn/1
  Uslow Dynam/1 -> I USLOW +/1(V)
  Iapp/1 -> Add/2
  gup/1 -> I USLOW +/2(a)
  dsm/1 -> I SLOW -/3(d)
  gsm/1 -> I SLOW -/2(a)
  dup/1 -> I USLOW +/3(d)

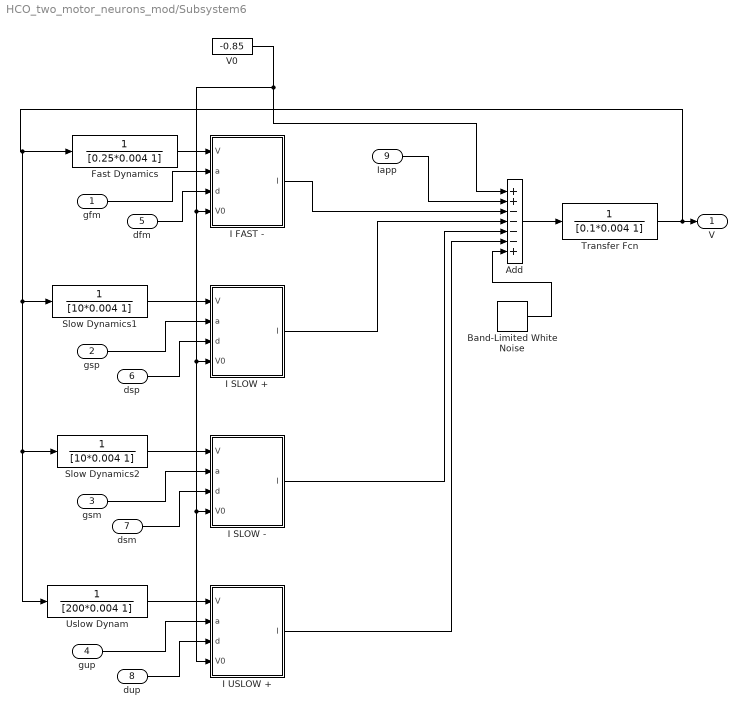
== system HCO_two_motor_neurons_mod/Subsystem6 ==
  gfm : Inport
  gsp : Inport  Port=2
  gsm : Inport  Port=3
  gup : Inport  Port=4
  dfm : Inport  Port=5
  dsp : Inport  Port=6
  dsm : Inport  Port=7
  dup : Inport  Port=8
  Iapp : Inport  Port=9
  Add : Sum  Inputs=++----+
  Band-Limited White Noise : simulink/Sources/Band-Limited White Noise  Cov=[noisePwr]  Ts=0.001  seed=floor(rand(1)*250000)
  Fast Dynamics : TransferFcn  Denominator=[0.25*0.004 1]
  I FAST - : MATLAB Function  TreatAsAtomicUnit=on
  I SLOW + : MATLAB Function  TreatAsAtomicUnit=on
  I SLOW - : MATLAB Function  TreatAsAtomicUnit=on
  I USLOW + : MATLAB Function  TreatAsAtomicUnit=on
  Slow Dynamics1 : TransferFcn  Denominator=[10*0.004 1]
  Slow Dynamics2 : TransferFcn  Denominator=[10*0.004 1]
  Transfer Fcn : TransferFcn  Denominator=[0.1*0.004 1]
  Uslow Dynam : TransferFcn  Denominator=[200*0.004 1]
  V0 : Constant  Value=-0.85
  V : Outport
  wires:
  dup/1 -> I USLOW +/3(d)
  gsm/1 -> I SLOW -/2(a)
  dsm/1 -> I SLOW -/3(d)
  gup/1 -> I USLOW +/2(a)
  Iapp/1 -> Add/2
  Uslow Dynam/1 -> I USLOW +/1(V)
  Add/1 -> Transfer Fcn/1
  Slow Dynamics1/1 -> I SLOW +/1(V)
  Slow Dynamics2/1 -> I SLOW -/1(V)
  I FAST -/1(I) -> Add/3
  I USLOW +/1(I) -> Add/6
  V0/1 -> I USLOW +/4(V0), I SLOW -/4(V0), I SLOW +/4(V0), I FAST -/4(V0), Add/1
  dsp/1 -> I SLOW +/3(d)
  gsp/1 -> I SLOW +/2(a)
  dfm/1 -> I FAST -/3(d)
  gfm/1 -> I FAST -/2(a)
  Fast Dynamics/1 -> I FAST -/1(V)
  I SLOW -/1(I) -> Add/5
  Transfer Fcn/1 -> Uslow Dynam/1, Slow Dynamics2/1, Slow Dynamics1/1, Fast Dynamics/1, V/1
  I SLOW +/1(I) -> Add/4
  Band-Limited White Noise/1 -> Add/7

== matlab function HCO_two_motor_neurons_mod/Subsystem1/I FAST - ==
  data: V input; I output; a input; d input; V0 input
function I = fcn(V,a,d,V0)

I = a*(tanh(V-d)-tanh(V0-d));

== matlab function HCO_two_motor_neurons_mod/HCO 1->1 ==
  data: V input; I output; gsyn input; d input
function I = fcn(V,gsyn,d)

I = gsyn*(tanh(2*(V-d))+1)/2;

== matlab function HCO_two_motor_neurons_mod/Mod Neuron1/I USLOW + ==
  data: V input; I output; a input; d input; V0 input
function I = fcn(V,a,d,V0)

I = a*(tanh(V-d)-tanh(V0-d));

== matlab function HCO_two_motor_neurons_mod/synapse 1->2 ==
  data: V input; I output; gsyn input; d input
function I = fcn(V,gsyn,d)

I = gsyn*(tanh(2*(V-d))+1)/2;

== matlab function HCO_two_motor_neurons_mod/Mod Neuron/I SLOW + ==
  data: V input; I output; a input; d input; V0 input
function I = fcn(V,a,d,V0)

I = a*(tanh(V-d)-tanh(V0-d));

== matlab function HCO_two_motor_neurons_mod/Mod Neuron/I SLOW - ==
  data: V input; I output; a input; d input; V0 input
function I = fcn(V,a,d,V0)

I = a*(tanh(V-d)-tanh(V0-d));

== matlab function HCO_two_motor_neurons_mod/Mod Neuron/I USLOW + ==
  data: V input; I output; a input; d input; V0 input
function I = fcn(V,a,d,V0)

I = a*(tanh(V-d)-tanh(V0-d));

== matlab function HCO_two_motor_neurons_mod/Sensory Return p ==
  data: u input; du input; y output; bar_amp input; buff_amp input
function y = fcn(u, du, bar_amp, buff_amp)

yu = tanh( 20*(cos(bar_amp+buff_amp)-cos(u)) );
ydu = (tanh(10*(du+0.1)) - tanh(10*(du-0.1)))/2 - 1;
y = yu + ydu;

== matlab function HCO_two_motor_neurons_mod/Sensory Return m ==
  data: u input; du input; y output; bar_amp input; buff_amp input
function y = fcn(u, du, bar_amp, buff_amp)

yu = tanh( 20*(cos(u)-cos(bar_amp-buff_amp)) );
ydu = (tanh(10*(du+0.1)) - tanh(10*(du-0.1)))/2 - 1;
y = yu + ydu;

== matlab function HCO_two_motor_neurons_mod/AngleToCurrent1 ==
  data: u input; y output; du input
function y = fcn(u, du)
uy = (1-tanh(15*(sin(u)-0.05)))/2 - 1;
duy = (tanh(5*(du+0.5)) - tanh(5*(du-0.5)))/2;
y = uy + duy;

== matlab function HCO_two_motor_neurons_mod/HCO 1->2 ==
  data: V input; I output; gsyn input; d input
function I = fcn(V,gsyn,d)

I = gsyn*(tanh(2*(V-d))+1)/2;

== matlab function HCO_two_motor_neurons_mod/Subsystem1/I SLOW + ==
  data: V input; I output; a input; d input; V0 input
function I = fcn(V,a,d,V0)

I = a*(tanh(V-d)-tanh(V0-d));

== matlab function HCO_two_motor_neurons_mod/HCO 1->3 ==
  data: V input; I output; gsyn input; d input
function I = fcn(V,gsyn,d)

I = gsyn*(tanh(2*(V-d))+1)/2;

== matlab function HCO_two_motor_neurons_mod/HCO 1->4 ==
  data: V input; I output; gsyn input; d input
function I = fcn(V,gsyn,d)

I = gsyn*(tanh(2*(V-d))+1)/2;

== matlab function HCO_two_motor_neurons_mod/Subsystem6/I FAST - ==
  data: V input; I output; a input; d input; V0 input
function I = fcn(V,a,d,V0)

I = a*(tanh(V-d)-tanh(V0-d));

== matlab function HCO_two_motor_neurons_mod/Subsystem6/I SLOW + ==
  data: V input; I output; a input; d input; V0 input
function I = fcn(V,a,d,V0)

I = a*(tanh(V-d)-tanh(V0-d));

== matlab function HCO_two_motor_neurons_mod/Subsystem6/I SLOW - ==
  data: V input; I output; a input; d input; V0 input
function I = fcn(V,a,d,V0)

I = a*(tanh(V-d)-tanh(V0-d));

== matlab function HCO_two_motor_neurons_mod/Subsystem6/I USLOW + ==
  data: V input; I output; a input; d input; V0 input
function I = fcn(V,a,d,V0)

I = a*(tanh(V-d)-tanh(V0-d));

== matlab function HCO_two_motor_neurons_mod/3 ==
  data: u input; y output; du input
function y = fcn(u, du)
uy = (1+tanh(15*(sin(u)+0.05)))/2 - 1;
duy = (tanh(5*(du+0.5)) - tanh(5*(du-0.5)))/2;
y = uy + duy;

== matlab function HCO_two_motor_neurons_mod/AngleToCurrent3 ==
  data: u input; y output; du input
function y = fcn(u, du)
uy = (1-tanh(15*(sin(u)-0.05)))/2 - 1;
duy = (tanh(5*(du+0.5)) - tanh(5*(du-0.5)))/2;
y = uy + duy;

== matlab function HCO_two_motor_neurons_mod/Mod Neuron4/I FAST - ==
  data: V input; I output; a input; d input; V0 input
function I = fcn(V,a,d,V0)

I = a*(tanh(V-d)-tanh(V0-d));

== matlab function HCO_two_motor_neurons_mod/Mod Neuron4/I SLOW + ==
  data: V input; I output; a input; d input; V0 input
function I = fcn(V,a,d,V0)

I = a*(tanh(V-d)-tanh(V0-d));

== matlab function HCO_two_motor_neurons_mod/Mod Neuron4/I SLOW - ==
  data: V input; I output; a input; d input; V0 input
function I = fcn(V,a,d,V0)

I = a*(tanh(V-d)-tanh(V0-d));

== matlab function HCO_two_motor_neurons_mod/Subsystem1/I SLOW - ==
  data: V input; I output; a input; d input; V0 input
function I = fcn(V,a,d,V0)

I = a*(tanh(V-d)-tanh(V0-d));

== matlab function HCO_two_motor_neurons_mod/Mod Neuron4/I USLOW + ==
  data: V input; I output; a input; d input; V0 input
function I = fcn(V,a,d,V0)

I = a*(tanh(V-d)-tanh(V0-d));

== matlab function HCO_two_motor_neurons_mod/Mod Neuron5/I FAST - ==
  data: V input; I output; a input; d input; V0 input
function I = fcn(V,a,d,V0)

I = a*(tanh(V-d)-tanh(V0-d));

== matlab function HCO_two_motor_neurons_mod/Mod Neuron5/I SLOW + ==
  data: V input; I output; a input; d input; V0 input
function I = fcn(V,a,d,V0)

I = a*(tanh(V-d)-tanh(V0-d));

== matlab function HCO_two_motor_neurons_mod/Mod Neuron5/I SLOW - ==
  data: V input; I output; a input; d input; V0 input
function I = fcn(V,a,d,V0)

I = a*(tanh(V-d)-tanh(V0-d));

== matlab function HCO_two_motor_neurons_mod/Mod Neuron5/I USLOW + ==
  data: V input; I output; a input; d input; V0 input
function I = fcn(V,a,d,V0)

I = a*(tanh(V-d)-tanh(V0-d));

== matlab function HCO_two_motor_neurons_mod/Sensory Return m2 ==
  data: u input; du input; y output; bar_amp input; buff_amp input
function y = fcn(u, du, bar_amp, buff_amp)

yu = tanh( 20*(cos(u)-cos(bar_amp-buff_amp)) );
ydu = (tanh(10*(du+0.1)) - tanh(10*(du-0.1)))/2 - 1;
y = yu + ydu;

== matlab function HCO_two_motor_neurons_mod/Sensory Return p2 ==
  data: u input; du input; y output; bar_amp input; buff_amp input
function y = fcn(u, du, bar_amp, buff_amp)

yu = tanh( 20*(cos(bar_amp+buff_amp)-cos(u)) );
ydu = (tanh(10*(du+0.1)) - tanh(10*(du-0.1)))/2 - 1;
y = yu + ydu;

== matlab function HCO_two_motor_neurons_mod/Subsystem4/I FAST - ==
  data: V input; I output; a input; d input; V0 input
function I = fcn(V,a,d,V0)

I = a*(tanh(V-d)-tanh(V0-d));

== matlab function HCO_two_motor_neurons_mod/Subsystem4/I SLOW + ==
  data: V input; I output; a input; d input; V0 input
function I = fcn(V,a,d,V0)

I = a*(tanh(V-d)-tanh(V0-d));

== matlab function HCO_two_motor_neurons_mod/Subsystem4/I SLOW - ==
  data: V input; I output; a input; d input; V0 input
function I = fcn(V,a,d,V0)

I = a*(tanh(V-d)-tanh(V0-d));

== matlab function HCO_two_motor_neurons_mod/Subsystem1/I USLOW + ==
  data: V input; I output; a input; d input; V0 input
function I = fcn(V,a,d,V0)

I = a*(tanh(V-d)-tanh(V0-d));

== matlab function HCO_two_motor_neurons_mod/Subsystem4/I USLOW + ==
  data: V input; I output; a input; d input; V0 input
function I = fcn(V,a,d,V0)

I = a*(tanh(V-d)-tanh(V0-d));

== matlab function HCO_two_motor_neurons_mod/Subsystem5/I FAST - ==
  data: V input; I output; a input; d input; V0 input
function I = fcn(V,a,d,V0)

I = a*(tanh(V-d)-tanh(V0-d));

== matlab function HCO_two_motor_neurons_mod/Subsystem5/I SLOW + ==
  data: V input; I output; a input; d input; V0 input
function I = fcn(V,a,d,V0)

I = a*(tanh(V-d)-tanh(V0-d));

== matlab function HCO_two_motor_neurons_mod/Subsystem5/I SLOW - ==
  data: V input; I output; a input; d input; V0 input
function I = fcn(V,a,d,V0)

I = a*(tanh(V-d)-tanh(V0-d));

== matlab function HCO_two_motor_neurons_mod/Subsystem5/I USLOW + ==
  data: V input; I output; a input; d input; V0 input
function I = fcn(V,a,d,V0)

I = a*(tanh(V-d)-tanh(V0-d));

== matlab function HCO_two_motor_neurons_mod/synapse 1->5 ==
  data: V input; I output; gsyn input; d input
function I = fcn(V,gsyn,d)

I = gsyn*(tanh(2*(V-d))+1)/2;

== matlab function HCO_two_motor_neurons_mod/synapse 1->6 ==
  data: V input; I output; gsyn input; d input
function I = fcn(V,gsyn,d)

I = gsyn*(tanh(2*(V-d))+1)/2;

== matlab function HCO_two_motor_neurons_mod/synapse 1->1 ==
  data: V input; I output; gsyn input; d input
function I = fcn(V,gsyn,d)

I = gsyn*(tanh(2*(V-d))+1)/2;

== matlab function HCO_two_motor_neurons_mod/Mod Neuron/I FAST - ==
  data: V input; I output; a input; d input; V0 input
function I = fcn(V,a,d,V0)

I = a*(tanh(V-d)-tanh(V0-d));

== matlab function HCO_two_motor_neurons_mod/1 ==
  data: u input; y output; du input
function y = fcn(u, du)
uy = (1+tanh(15*(sin(u)+0.05)))/2 - 1;
duy = (tanh(5*(du+0.5)) - tanh(5*(du-0.5)))/2;
y = uy + duy;

== matlab function HCO_two_motor_neurons_mod/Mod Neuron1/I FAST - ==
  data: V input; I output; a input; d input; V0 input
function I = fcn(V,a,d,V0)

I = a*(tanh(V-d)-tanh(V0-d));

== matlab function HCO_two_motor_neurons_mod/Mod Neuron1/I SLOW + ==
  data: V input; I output; a input; d input; V0 input
function I = fcn(V,a,d,V0)

I = a*(tanh(V-d)-tanh(V0-d));

== matlab function HCO_two_motor_neurons_mod/Mod Neuron1/I SLOW - ==
  data: V input; I output; a input; d input; V0 input
function I = fcn(V,a,d,V0)

I = a*(tanh(V-d)-tanh(V0-d));
